simulink model "global_positions"  (R2023b)
settings: Solver=VariableStepAuto  StartTime=0.0  StopTime=25  RelTol=1e-3
values from neighbouring files (symbols this model uses):
  A = [0 1 0 0 ... (first row only)    [Amatrix.m]    (also in task2_init.m; task2_plot.m = Amatrix(m,Vx,cf,cr,lf,lr,Iz))
  A1 = [0 1 0 0 ... (first row only)    [task2_init.m]    (also in task2_plot.m = A1matrix(m,Vx,cf,cr,lf,lr,Iz))
  amplitude = pi/6    (= 0.523598775598)    [task1_plot.m]    (also in task2_plot.m)
  B = [0 ... (first row only)    [Bmatrix.m]    (also in task2_init.m; task2_plot.m = Bmatrix(m,cf,Iz))
  B1 = [B1_1 B_d]    [task2_init.m]    (also in task2_plot.m)
  C = eye (4)    [task2_init.m]    (also in task2_plot.m = eye(4))
  C1 = eye (4)    [task2_init.m]    (also in task2_plot.m = eye(4))
  D = zeros(4,4)    [task2_init.m]    (also in task2_plot.m = zeros(4,1))
  D1 = zeros(4,2)    [task2_init.m]    (also in task2_plot.m)
  delta_ff = feedforward(m, Vx, lf, lr, cf, cr, r, Kpp)    [task2_plot.m]
  frequency = 0.5    [task1_plot.m]    (also in task2_plot.m)
  Kpp = place(A1,B1_1,P)    [task2_plot.m]
  psidot_des = Vx/r    (= 0.0194444444444)    [task2_plot.m]
  Vx = (velocity * 1000) / 3600    (= 8.33333333333)    [task1_plot.m]    (also in task2_plot.m = 19.4444444444)
  x2_0 = zeros (4,1)+2    [task2_plot.m]
  x_0 = zeros(4,1)    [task2_plot.m]
settings Model: Creator=seuffoakouanhangoume  LastModifiedBy=seuffoakouanhangoume
settings OptimizationCC: BlockReduction=off  DefaultParameterBehavior=Inlined  BufferReuse=off

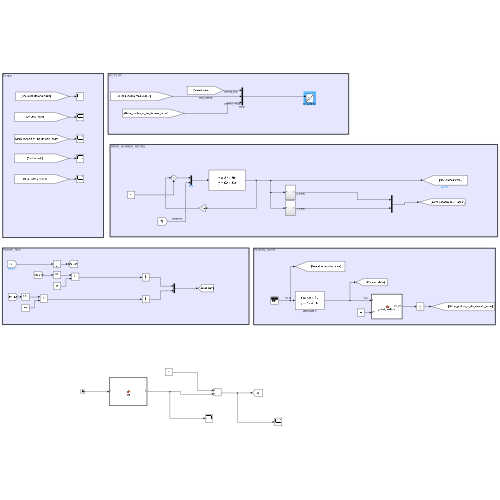
[thumbnail: Simulink's stored preview of the top-level diagram]
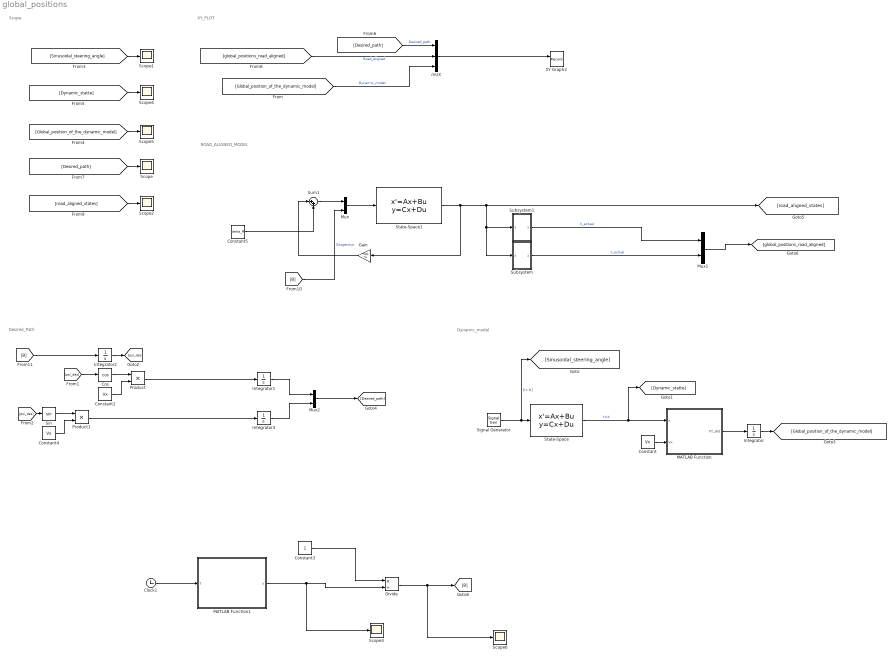
== system global_positions ==
  note: ROAD_ALIGNED_MODEL
  note: XY_PLOT
  note: Desired_Path
  note: Dynamic_model
  note: Scope
  Clock1 : Clock
  Constant : Constant  Value=Vx
  Constant2 : Constant  Value=Vx
  Constant3 : Constant
  Constant4 : Constant  Value=Vx
  Constant5 : Constant  Value=delta_ff
  Cos : Trigonometry  Operator=cos
  Divide : Product  Inputs=*/
  Gain : Gain  Gain=-Kpp  Multiplication=Matrix(K*u)
  Integrator{,1..3} (4 alike) : Integrator
  MATLAB Function : MATLAB Function  TreatAsAtomicUnit=on
  MATLAB Function1 : MATLAB Function  TreatAsAtomicUnit=on
  Mux : Mux  Inputs=2
  Mux1 : Mux  Inputs=2
  Mux2 : Mux  Inputs=2
  Product : Product
  Product1 : Product
  Scope{,1..6} (7 alike) : Scope
  Signal Generator : SignalGenerator  Amplitude=amplitude  Frequency=frequency
  Sin : Trigonometry
  State-Space : StateSpace  A=A  B=B  C=C  D=D  InitialCondition=x_0
  State-Space1 : StateSpace  A=A1  B=B1  C=C1  D=D1  InitialCondition=x2_0
  Subsystem : Subsystem
  Subsystem1 : Subsystem
  Sum1 : Sum  Inputs=|++
  XY Graph2 : Record  FileSettingsInternal="{\"entries\":[{\"content\":{\"excelSettings\":{\"content\":{},\"type\":\"Streamout.ExcelSettings\"}},\"type\":\"Streamout.FileSettingStorage\",\"uuid\":\"\"}],\"packageUris\":[\"http:\\/\\/schema.mathworks.com\\/mf0\\/streamout_blocks\\/R2020a\"],\"version\":\"1.0\"}"  Layout=[1 1]  SignalsInternal="{\"entries\":[{\"content\":{\"signals\":[{\"content\":{\"blockPath\":[],\"dimensions\":[6,1],\"domain\":\"\",\"hasChildren\":true,\"lineColor\":\"#64d413\",\"port\":1,\"sid\":[\"\"],\"signalID\":6455,\"signalName\":\"mUX\"},\"type\":\"RecordBlkView.Signal\",\"uuid\":\"\"},{\"content\":{\"blockPath\":[],\"channel\":[1,1],\"dimensions\":[6,1],\"domain\":\"\",\"lineColor\":\"#22b573\",\"parentID\":6455,\"plots\":[1],\"port\":1,\"sid\":[\"\"],\"signalID\":6456,\"signalName\":\"mUX\"},\"type\":\"RecordBlkView.Signal\",\"uuid\":\"\"},{\"content\":{\"blockPath\":[],\"dimensions\":[1],\"domain\":\"\",\"lineColor\":\"#0072bd\",\"port\":2,\"sid\":[\"\"],\"signalID\":6460},\"type\":\"RecordBlkView.Signal\",\"uuid\":\"\"},{\"content\":{\"blockPath\":[],\"channel\":[2,1],\"dimensions\":[6,1],\"domain\":\"\",\"lineColor\":\"#d95319\",\"parentID\":6455,\"plots\":[1],\"port\":1,\"sid\":[\"\"],\"signalID\":6464,\"signalName\":\"mUX\"},\"type\":\"RecordBlkView.Signal\",\"uuid\":\"\"},{\"content\":{\"blockPath\":[],\"channel\":[3,1],\"dimensions\":[6,1],\"domain\":\"\",\"lineColor\":\"#edb120\",\"parentID\":6455,\"port\":1,\"sid\":[\"\"],\"signalID\":6465,\"signalName\":\"mUX\"},\"type\":\"RecordBlkView.Signal\",\"uuid\":\"\"},{\"content\":{\"blockPath\":[],\"channel\":[4,1],\"dimensions\":[6,1],\"domain\":\"\",\"lineColor\":\"#7e2f8e\",\"parentID\":6455,\"plots\":[1],\"port\":1,\"sid\":[\"\"],\"signalID\":6466,\"signalName\":\"mUX\"},\"type\":\"RecordBlkView.Signal\",\"uuid\":\"\"},{\"content\":{\"blockPath\":[],\"channel\":[5,1],\"dimensions\":[6,1],\"domain\":\"\",\"lineColor\":\"#77ac30\",\"parentID\":6455,\"port\":1,\"sid\":[\"\"],\"signalID\":6467,\"signalName\":\"mUX\"},\"type\":\"RecordBlkView.Signal\",\"uuid\":\"\"},{\"content\":{\"blockPath\":[],\"channel\":[6,1],\"dimensions\":[6,1],\"domain\":\"\",\"lineColor\":\"#4dbeee\",\"parentID\":6455,\"port\":1,\"sid\":[\"\"],\"signalID\":6468,\"signalName\":\"mUX\"},\"type\":\"RecordBlkView.Signal\",\"uuid\":\"\"}]},\"type\":\"RecordBlkView.InputSignals\",\"uuid\":\"\"}],\"packageUris\":[\"http:\\/\\/schema.mathworks.com\\/mf0\\/streamout_blocks\\/R2020a\"],\"version\":\"1.0\"}"  VisualizationBindings="{\"xyplotplugin\":{\"info\":[{\"series\":[{\"bindingParametersList\":[{\"parameter\":\"Y-Axis\",\"signalID\":6466,\"signalName\":\"mUX(4,1)\"}],\"seriesID\":583},{\"bindingParametersList\":[{\"parameter\":\"X-Axis\",\"signalID\":6456,\"signalName\":\"mUX(1,1)\"},{\"parameter\":\"Y-Axis\",\"signalID\":6464,\"signalName\":\"mUX(2,1)\"}],\"seriesID\":90}],\"subplotID\":1}]}}"  CompatibilityTag=XY  st=-1
  mUX : Mux  Inputs=3
  wires:
  Product1/1 -> Integrator3/1
  State-Space1/1 -> Gain/1, [road_aligned_states], Subsystem/1(x), Subsystem1/1(x)
  Cos/1 -> Product/1
  Subsystem/1(Out1) -> Mux1/2  "Y_actual"
  [psi_des] -> Sin/1
  [B] -> Integrator2/1
  Sin/1 -> Product1/1
  [Global_position_of_the_dynamic_model] -> mUX/3  "Dynamic_model"
  Constant2/1 -> Product/2
  State-Space/1 -> [Dynamic_statte], MATLAB Function/1(x)  "Y=X"
  [B] -> Mux/2  "Exogenous"
  Constant4/1 -> Product1/2
  Mux1/1 -> [global_positions_road_aligned]
  Subsystem1/1(Out1) -> Mux1/1  "X_actual"
  mUX/1 -> XY Graph2/1
  Integrator/1 -> [Global_position_of_the_dynamic_model]
  Integrator2/1 -> [psi_des]
  [psi_des] -> Cos/1
  MATLAB Function/1(XY_dot) -> Integrator/1
  Constant/1 -> MATLAB Function/2(Vx)
  Signal Generator/1 -> [Sinusoidal_steering_angle], State-Space/1  "[U; D]"
  [Sinusoidal_steering_angle] -> Scope1/1
  [Dynamic_statte] -> Scope4/1
  [Global_position_of_the_dynamic_model] -> Scope5/1
  Product/1 -> Integrator1/1
  Integrator1/1 -> Mux2/1
  [Desired_path] -> mUX/1  "Desired_path"
  [Desired_path] -> Scope/1
  [global_positions_road_aligned] -> mUX/2  "Road_aligned"
  [road_aligned_states] -> Scope2/1
  Integrator3/1 -> Mux2/2
  Mux2/1 -> [Desired_path]
  Mux/1 -> State-Space1/1
  Constant5/1 -> Sum1/2
  Sum1/1 -> Mux/1
  Gain/1 -> Sum1/1
  Clock1/1 -> MATLAB Function1/1(t)
  MATLAB Function1/1(y) -> Scope3/1, Divide/2
  Constant3/1 -> Divide/1
  Divide/1 -> Scope6/1, [B]

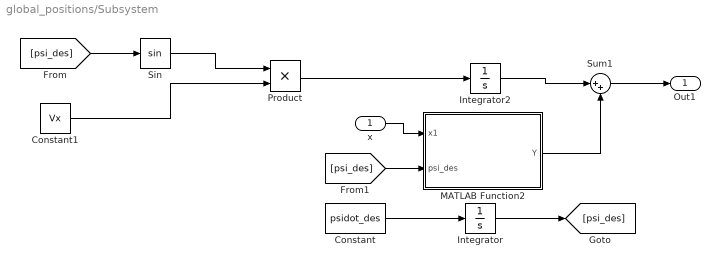
== system global_positions/Subsystem ==
  x : Inport
  Constant : Constant  Value=psidot_des
  Constant1 : Constant  Value=Vx
  Integrator : Integrator
  Integrator2 : Integrator
  MATLAB Function2 : MATLAB Function  TreatAsAtomicUnit=on
  Product : Product
  Sin : Trigonometry
  Sum1 : Sum  Inputs=|++
  Out1 : Outport
  wires:
  Sum1/1 -> Out1/1
  Integrator/1 -> [psi_des]
  MATLAB Function2/1(Y) -> Sum1/2
  x/1 -> MATLAB Function2/1(x1)
  Constant/1 -> Integrator/1
  [psi_des] -> MATLAB Function2/2(psi_des)
  Integrator2/1 -> Sum1/1
  Product/1 -> Integrator2/1
  [psi_des] -> Sin/1
  Sin/1 -> Product/1
  Constant1/1 -> Product/2

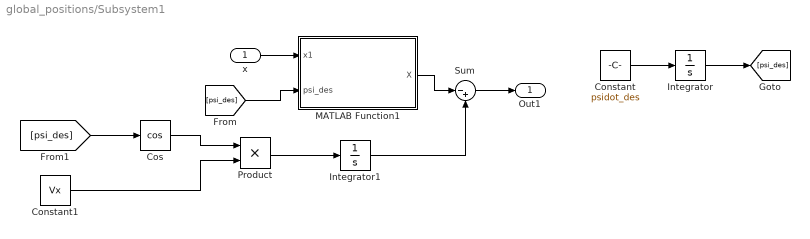
== system global_positions/Subsystem1 ==
  x : Inport
  Constant : Constant  Value=psidot_des
  Constant1 : Constant  Value=Vx
  Cos : Trigonometry  Operator=cos
  Integrator : Integrator
  Integrator1 : Integrator
  MATLAB Function1 : MATLAB Function  TreatAsAtomicUnit=on
  Product : Product
  Sum : Sum  Inputs=|-+
  Out1 : Outport
  wires:
  Sum/1 -> Out1/1
  [psi_des] -> MATLAB Function1/2(psi_des)
  Integrator1/1 -> Sum/2
  MATLAB Function1/1(X) -> Sum/1
  x/1 -> MATLAB Function1/1(x1)
  Constant/1 -> Integrator/1
  Integrator/1 -> [psi_des]
  [psi_des] -> Cos/1
  Constant1/1 -> Product/2
  Cos/1 -> Product/1
  Product/1 -> Integrator1/1

== matlab function global_positions/Subsystem1/MATLAB Function1 ==
  data: x1 input; X output; psi_des input
function X = func2(x1,psi_des)

X = x1(1)*sin(psi_des);

end

== matlab function global_positions/MATLAB Function ==
  data: x input; XY_dot output; Vx input
function XY_dot = global_positions(x,Vx)
XY_dot = [Vx*cos(x(3))+x(2)*sin(x(3)) ;
      x(2)*cos(x(3))+Vx*sin(x(3))];

end

== matlab function global_positions/Subsystem/MATLAB Function2 ==
  data: x1 input; Y output; psi_des input
function Y = fuc1(x1,psi_des)

Y = x1(1)*cos(psi_des);

end

== matlab function global_positions/MATLAB Function1 ==
  data: t input; y output
function y = fcn(t)
    if t >= 10
        y = 1000;
    else
        y = inf;
    end
